simulink model "preg"  (R2021b)
settings: Solver=VariableStepAuto  StartTime=0.0  StopTime=5  RelTol=1e-3
undefined symbols (not defined in the file): Angeln, J, ke, km, Kn, L, Moth, R, U
settings Model: Creator=vital  LastModifiedBy=vital
settings SolverCC: AlgebraicLoopSolver=TrustRegion
settings DebuggingCC: SFMachineParentedDataDiag=warning

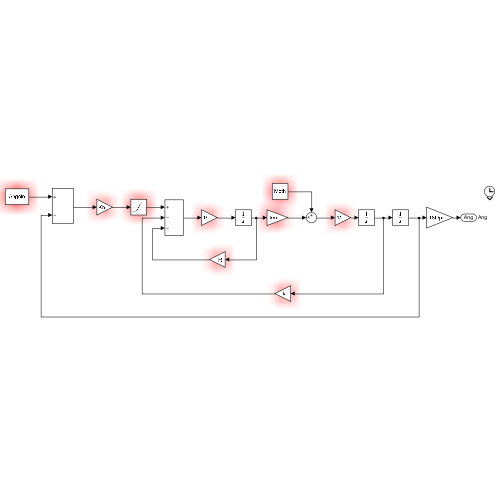
[thumbnail: Simulink's stored preview of the top-level diagram]
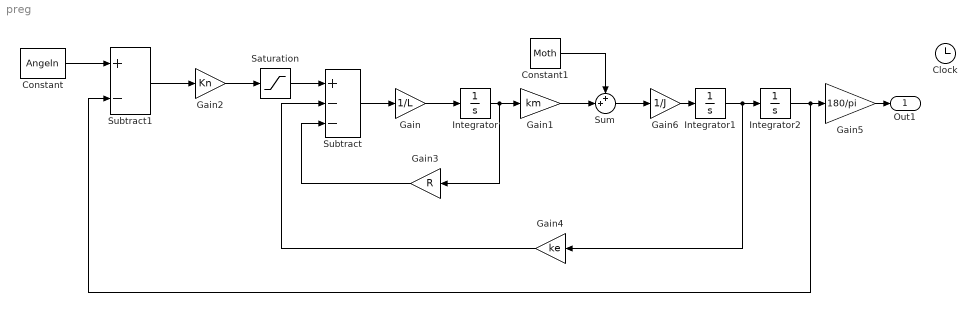
== system preg ==
  Clock : Clock
  Constant : Constant  Value=Angeln
  Constant1 : Constant  Value=Moth
  Gain : Gain  Gain=1/L
  Gain1 : Gain  Gain=km
  Gain2 : Gain  Gain=Kn
  Gain3 : Gain  Gain=R
  Gain4 : Gain  Gain=ke
  Gain5 : Gain  Gain=180/pi
  Gain6 : Gain  Gain=1/J
  Integrator : Integrator
  Integrator1 : Integrator
  Integrator2 : Integrator
  Saturation : Saturate  UpperLimit=U  LowerLimit=-U
  Subtract : Sum  Inputs=+--
  Subtract1 : Sum  Inputs=+-
  Sum : Sum  Inputs=++|
  Out1 : Outport  SignalName=Ang
  wires:
  Subtract/1 -> Gain/1
  Gain/1 -> Integrator/1
  Gain2/1 -> Saturation/1
  Integrator/1 -> Gain1/1, Gain3/1
  Gain3/1 -> Subtract/3
  Integrator1/1 -> Gain4/1, Integrator2/1
  Gain4/1 -> Subtract/2
  Saturation/1 -> Subtract/1
  Constant/1 -> Subtract1/1
  Gain5/1 -> Out1/1
  Integrator2/1 -> Subtract1/2, Gain5/1
  Subtract1/1 -> Gain2/1
  Gain6/1 -> Integrator1/1
  Sum/1 -> Gain6/1
  Gain1/1 -> Sum/2
  Constant1/1 -> Sum/1
